simulink model "modC"  (R2023a)
settings: Solver=VariableStepAuto  StartTime=0.0  StopTime=10.0  RelTol=1e-3
libraries: simulink x2
settings Model: Creator=Francesco  LastModifiedBy=Francesco

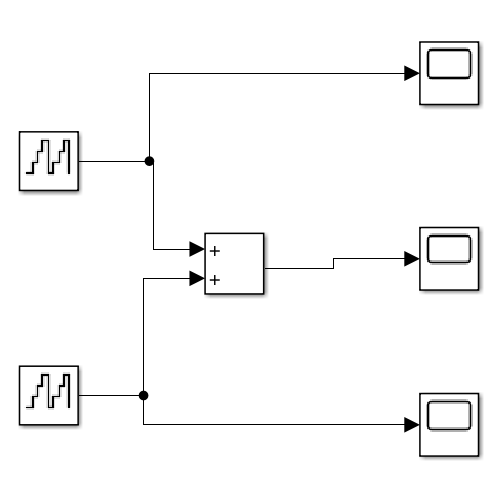
[thumbnail: Simulink's stored preview of the top-level diagram]
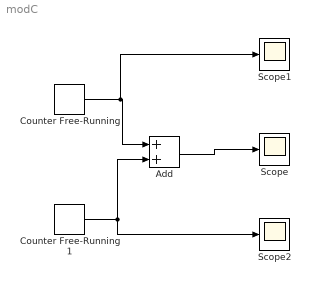
== system modC ==
  Add : Sum
  Counter Free-Running : simulink/Sources/Counter Free-Running  NumBits=16  tsamp=-1
  Counter Free-Running1 : simulink/Sources/Counter Free-Running  NumBits=8  tsamp=-1
  Scope : Scope
  Scope1 : Scope
  Scope2 : Scope
  wires:
  Counter Free-Running/1 -> Scope1/1, Add/1
  Counter Free-Running1/1 -> Add/2, Scope2/1
  Add/1 -> Scope/1
